simulink model "GPSSmoothingEstimation"  (R2018a)
settings: Solver=VariableStepAuto  StartTime=0.0  StopTime=10.0  RelTol=1e-3
undefined symbols (not defined in the file): magnitude, SkywalkerX8
libraries: sharedTrackingLibrary x1, dspmtrx3 x1
settings Model: Creator=David  LastModifiedBy=David

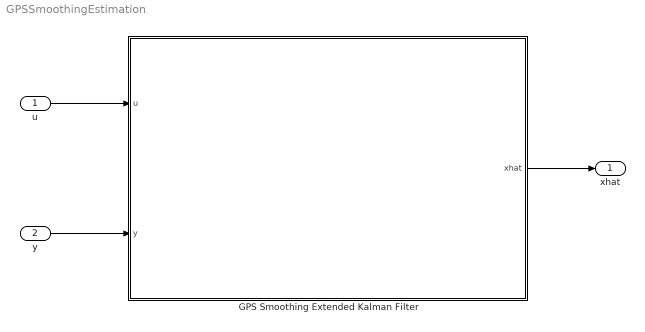
== system GPSSmoothingEstimation ==
  u : Inport  PortDimensions=5  SampleTime=SkywalkerX8.Sensors.EKF.GPSSmoothing.StateTransitionSampleTime
  y : Inport  Port=2  PortDimensions=6  SampleTime=SkywalkerX8.Sensors.EKF.GPSSmoothing.MeasurementSampleTime
  GPS Smoothing Extended Kalman Filter : Subsystem
      mask Display:
      | port_label('input', 1, '{\bf u} = [V_a, q, r, \Phi, \theta]', 'texMode', 'On')
      | port_label('input', 2, '{\bf y} = [y_{GPS_N}, y_{GPS_E}, y_{GPS_{V_g}}, y_{GPS_\chi}, y_{GPS_{wind_N}}, y_{GPS_{wind_E}}]', 'texMode', 'On')
      | 
      | port_label('output', 1, '{\bf x_{est}} = [p_n, p_e, V_g, \chi, w_n, w_e, \psi]', 'texMode', 'On')
  xhat : Outport
  wires:
  y/1 -> GPS Smoothing Extended Kalman Filter/2(y)
  u/1 -> GPS Smoothing Extended Kalman Filter/1(u)
  GPS Smoothing Extended Kalman Filter/1(xhat) -> xhat/1

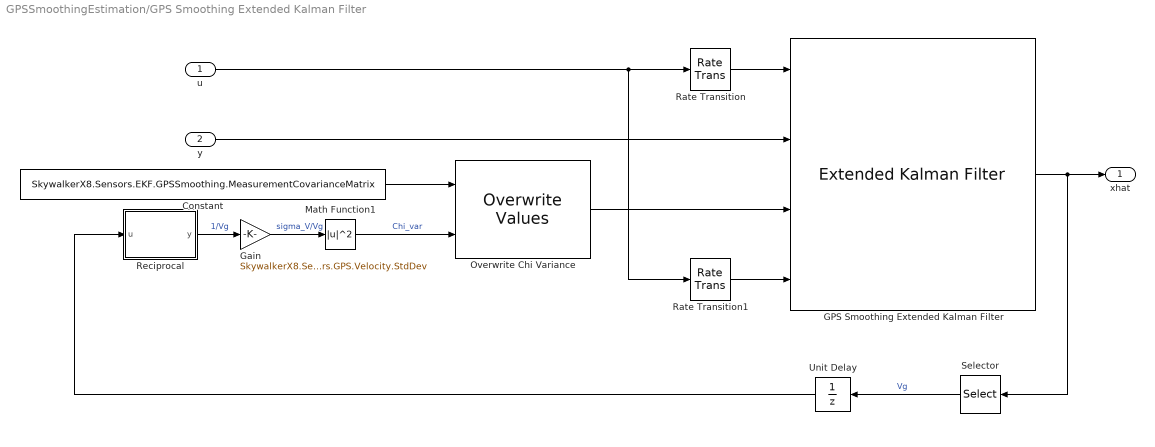
== system GPSSmoothingEstimation/GPS Smoothing Extended Kalman Filter ==
  u : Inport  PortDimensions=5
  y : Inport  Port=2  PortDimensions=6
  Constant : Constant  Value=SkywalkerX8.Sensors.EKF.GPSSmoothing.MeasurementCovarianceMatrix
  GPS Smoothing Extended Kalman Filter : sharedTrackingLibrary/Extended Kalman Filter  StateTransitionFcn=GPSSmoothingTransitionEstimate  HasStateTransitionJacobianFcn=on  StateTransitionJacobianFcn=GPSSmoothingTransitionEstimate_Jacobian  HasAdditiveProcessNoise=Additive  ProcessNoise=SkywalkerX8.Sensors.EKF.GPSSmoothing.ProcessCovarianceMatrix  HasTimeVaryingProcessNoise=off  HasStateTransitionFcnExtraArgument=1  InitialState=SkywalkerX8.Sensors.EKF.GPSSmoothing.InitialState  InitialStateCovariance=SkywalkerX8.Sensors.EKF.GPSSmoothing.InitialStateCovarianceMatrix  MeasurementFcn1=GPSSmoothingMeasurementEstimate  HasMeasurementJacobianFcn1=on  MeasurementJacobianFcn1=GPSSmoothingMeasurementEstimate_Jacobian  HasMeasurementEnablePort1=off  HasAdditiveMeasurementNoise1=Additive  MeasurementNoise1=SkywalkerX8.Sensors.EKF.GPSSmoothing.MeasurementCovarianceMatrix  HasTimeVaryingMeasurementNoise1=on  HasMeasurementFcnExtraArgument1=1  MeasurementFcn2=myMeasurementFcn  HasMeasurementJacobianFcn2=off  HasMeasurementEnablePort2=off  HasAdditiveMeasurementNoise2=Additive  MeasurementNoise2=1  HasTimeVaryingMeasurementNoise2=off  HasMeasurementFcnExtraArgument2=0  MeasurementFcn3=myMeasurementFcn  HasMeasurementJacobianFcn3=off  HasMeasurementEnablePort3=off  HasAdditiveMeasurementNoise3=Additive  MeasurementNoise3=1  HasTimeVaryingMeasurementNoise3=off  HasMeasurementFcnExtraArgument3=0  MeasurementFcn4=myMeasurementFcn  HasMeasurementJacobianFcn4=off  HasMeasurementEnablePort4=off  HasAdditiveMeasurementNoise4=Additive  MeasurementNoise4=1  HasTimeVaryingMeasurementNoise4=off  HasMeasurementFcnExtraArgument4=0  MeasurementFcn5=myMeasurementFcn  HasMeasurementJacobianFcn5=off  HasMeasurementEnablePort5=off  HasAdditiveMeasurementNoise5=Additive  MeasurementNoise5=1  HasTimeVaryingMeasurementNoise5=off  HasMeasurementFcnExtraArgument5=0  EnableMultirate=on  StateTransitionFcnSampleTime=SkywalkerX8.Sensors.EKF.GPSSmoothing.StateTransitionSampleTime  MeasurementFcn1SampleTime=SkywalkerX8.Sensors.EKF.GPSSmoothing.MeasurementSampleTime  MeasurementFcn2SampleTime=1  MeasurementFcn3SampleTime=1  MeasurementFcn4SampleTime=1  MeasurementFcn5SampleTime=1  UseCurrentEstimator=on  OutputStateCovariance=off  DataType=double  SampleTime=1  NumberOfMeasurements=1
      settings: SourceProductName=Control System Toolbox  SourceProductBaseCode=CT
  Gain : Gain  Gain=SkywalkerX8.Sensors.GPS.Velocity.StdDev
  Math Function1 : Math  Operator=magnitude^2  SaturateOnIntegerOverflow=on
  Overwrite Chi Variance : dspmtrx3/Overwrite Values  OverWriteDiag=Submatrix  valFrom2ndIP=Second input port  ConstValue=0  RowSpan=One row  RowStartMode=Index  RowStartIndex=4  RowEndMode=Last  RowEndIndex=1  ColSpan=One column  ColStartMode=First  ColStartIndex=1  ColEndMode=Last  ColEndIndex=1  DiagSpan=Range of elements  DiagStartMode=Index  DiagStartIndex=2  DiagEndMode=Index  DiagEndIndex=4
      settings: SourceProductName=DSP System Toolbox  SourceProductBaseCode=DS
  Rate Transition : RateTransition  OutPortSampleTime=SkywalkerX8.Sensors.EKF.GPSSmoothing.StateTransitionSampleTime
  Rate Transition1 : RateTransition  OutPortSampleTime=SkywalkerX8.Sensors.EKF.GPSSmoothing.MeasurementSampleTime
  Reciprocal : MATLAB Function  TreatAsAtomicUnit=on
  Selector : Selector  InputPortWidth=7  IndexOptions=Index vector (dialog)  Indices=3  OutputSizes=1
  Unit Delay : UnitDelay  InitialCondition=SkywalkerX8.Sensors.EKF.GPSSmoothing.InitialState(3)  SampleTime=SkywalkerX8.Sensors.EKF.GPSSmoothing.MeasurementSampleTime
  xhat : Outport
  wires:
  y/1 -> GPS Smoothing Extended Kalman Filter/2
  GPS Smoothing Extended Kalman Filter/1 -> Selector/1, xhat/1
  Reciprocal/1(y) -> Gain/1  "1/Vg"
  Gain/1 -> Math Function1/1  "sigma_V/Vg"
  Math Function1/1 -> Overwrite Chi Variance/2  "Chi_var"
  Constant/1 -> Overwrite Chi Variance/1
  Overwrite Chi Variance/1 -> GPS Smoothing Extended Kalman Filter/3
  u/1 -> Rate Transition1/1, Rate Transition/1
  Selector/1 -> Unit Delay/1  "Vg"
  Unit Delay/1 -> Reciprocal/1(u)
  Rate Transition/1 -> GPS Smoothing Extended Kalman Filter/1
  Rate Transition1/1 -> GPS Smoothing Extended Kalman Filter/4

== matlab function GPSSmoothingEstimation/GPS Smoothing Extended Kalman Filter/Reciprocal ==
  data: u input; y output
function y = reciprocal(u)

    if (u ~= 0)
       y = 1/u;
    else
       y = 1E06; 
    end

end
